simulink library "INT_EnvT_DD"  (R2016b)
settings: Solver=VariableStepAuto  StartTime=0.0  StopTime=10.0  RelTol=1e-3
settings Model: Creator=Administrator  LastModifiedBy=Administrator

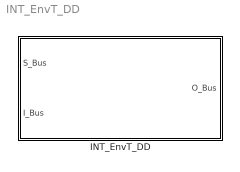
== system INT_EnvT_DD ==
  INT_EnvT_DD : Subsystem

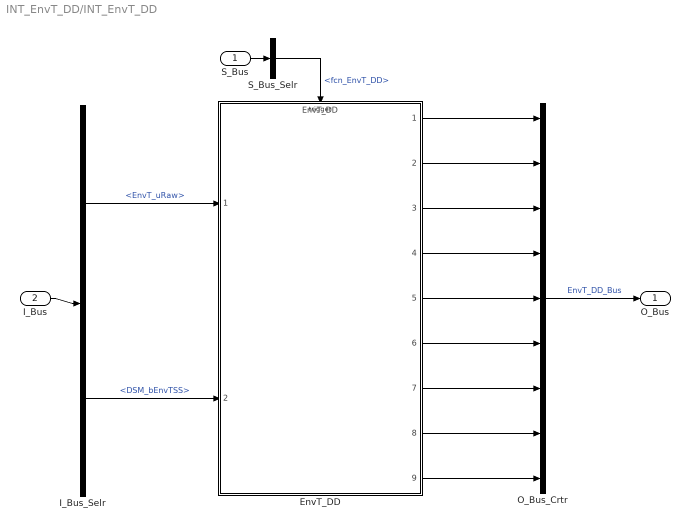
== system INT_EnvT_DD/INT_EnvT_DD ==
  S_Bus : Inport
  I_Bus : Inport  Port=2
  EnvT_DD : ModelReference  ModelNameDialog=EnvT_DD  SimulationMode=Normal  ModelReferenceVersion=1.11  TriggerPortName=function  TriggerPortTriggerType=function-call  TriggerPortStatesWhenEnabling=held
  I_Bus_Selr : BusSelector  OutputSignals=EnvT_uRaw,DSM_bEnvTSS
  O_Bus_Crtr : BusCreator  Inputs=9
  S_Bus_Selr : BusSelector  OutputSignals=fcn_EnvT_DD
  O_Bus : Outport
  wires:
  S_Bus_Selr/1 -> EnvT_DD/Trigger  "<fcn_EnvT_DD>"
  S_Bus/1 -> S_Bus_Selr/1
  I_Bus/1 -> I_Bus_Selr/1
  I_Bus_Selr/1 -> EnvT_DD/1  "<EnvT_uRaw>"
  I_Bus_Selr/2 -> EnvT_DD/2  "<DSM_bEnvTSS>"
  O_Bus_Crtr/1 -> O_Bus/1  "EnvT_DD_Bus"
  EnvT_DD/1 -> O_Bus_Crtr/1
  EnvT_DD/2 -> O_Bus_Crtr/2
  EnvT_DD/3 -> O_Bus_Crtr/3
  EnvT_DD/4 -> O_Bus_Crtr/4
  EnvT_DD/5 -> O_Bus_Crtr/5
  EnvT_DD/6 -> O_Bus_Crtr/6
  EnvT_DD/7 -> O_Bus_Crtr/7
  EnvT_DD/8 -> O_Bus_Crtr/8
  EnvT_DD/9 -> O_Bus_Crtr/9
